simulink library "kalmanlib"  (Simulink 7.0)
undefined symbols (not defined in the file): dt, P0, Q, seed1, tS, x0
libraries: kalmanlib x10, simulink x6
(part 1 of 2)
settings Model: Creator=peter  LastModifiedBy=peter  ExtModeAutoUpdateStatusClock=off

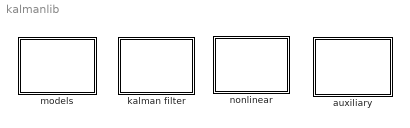
== system kalmanlib ==
  auxiliary : Subsystem
  kalman filter : Subsystem
  models : Subsystem
  nonlinear : Subsystem

== system kalmanlib/auxiliary ==
  Discrete Derivative : Subsystem  mask{x0=1, tS=0.01}
      mask prompts: x0 "Anfangs-Wert für x"; tS "Sample-Zeit"
      mask Display:
      | port_label('input', 1, 'x')
      | port_label('output', 1, 'v')
      | text(0.4, 0.7, 'd')
      | text(0.4, 0.4, 'dt')
      | plot([0.35 0.6], [0.5 0.5])
  Mean : Subsystem  mask{tS=1}
      mask prompts: tS "Sample-Zeit"
      mask Display: disp('total mean\n over time')
  Multivariate Normal  Distribution : Subsystem  mask(Multivariate Normal Distribution){m=0, P=Q, seed=seed1, tS=tS, C=0}
      mask prompts: m "Mean"; P "Covariance matrix"; seed "Initial seed"; tS "Sample time"; C "Root of P"
      mask help: Output a multivariate normally (Gaussian) distributed random signal.
      mask init:
      | [C, res] = sqrtm(P);
      mask Display: disp('N(m,P)')
  Osci : Subsystem
      settings: OpenFcn=open_system(find_system(gcbh, 'Name', 'Scope'), 'force')
  Variable Multivariate  Normal Distribution : Subsystem  mask(Multivariate Normal Distribution){m=0, seed=seed', tS=dt}
      mask prompts: m "Mean"; seed "Initial seed"; tS "Sample time"
      mask help: Output a multivariate normally (Gaussian) distributed random signal.
      mask Display:
      | port_label('input', 1, 'P')
      | port_label('output', 1, 'N(m,P)')

== system kalmanlib/kalman filter ==
  Extended Kalman Filter (Measurement) : Subsystem  mask(Kalman Filter){A=[1, 0, 1, 0, 0.5, 0; 0, 1, 0, 1, 0, 0.5;   0, 0, 1, 0, 1, 0; 0, 0, 0, 1, 0, 1;  0, 0, 0, 0, 1, 0;  0, 0, 0, 0, 0, 1], B=0, Q=[1 0 2 0 2 0; 0 1 0 2 0 2; 2 0 4 0 4 0; 0 2 0 4 0 4; 2 0 4 0 4 0; 0 2 0 4 0 4]*1e-4, R=[4 0; 0 4]*1e-4, x0=[40.254 25.117 0.492 0.112 -0.02 0.02]', P0=diag([100 100 1 1 0 0])*1e-6}
      mask prompts: A "Übertragungsmatrix A"; B "Kontrollmatrix B"; Q "Varianz der x-Störung Q"; R "Varianz der y-Störung R"; x0 "geschätzter Anfangsvektor x0"; P0 "geschätzte x-Anfangsvarianz P"
      mask Display:
      | disp('EKF (M)')
      | port_label('input', 1, 'u')
      | port_label('input', 2, 'z')
      | port_label('output', 1, 'x')
      | port_label('output', 2, 'P')
  Extended Kalman Filter (System) : Subsystem  mask(Extended Kalman Filter (A)){B=0, H=[1,0,0], Q=[0 0 0; 0 0 0; 0 0 0], R=[1e-3], x0=[1; 0; 0], P0=[1,0,0; 0,1,0; 0,0,10]*1e-2}
      mask prompts: B "Kontrollmatrix B"; H "Beobachtungsmatrix H"; Q "Varianz der x-Störung Q"; R "Varianz der y-Störung R"; x0 "geschätzter Anfangsvektor x0"; P0 "geschätzte x-Anfangsvarianz P"
      mask help: Extended Kalman Filter with a nonlinear system block, but linear control and measurement
      mask Display:
      | disp('EKF (A)')
      | port_label('input', 1, 'u')
      | port_label('input', 2, 'z')
      | port_label('output', 1, 'x')
      | port_label('output', 2, 'P')
  Kalman Filter : Subsystem  mask(Kalman Filter){A=[cos(0.01), sin(0.01); -sin(0.01), cos(0.01)], B=0, H=[1,0], Q=[0 0; 0 0], R=[2e-4], x0=[1; 0], P0=[10, 0; 0, 10]*1e-3}
      mask prompts: A "system matrix A"; B "control matrix B"; H "observation matrix H"; Q "variance of system noise Q"; R "variance of  measurement noise R"; x0 "estimated initial value x0"; P0 "estimated initial filter variance P0"
      mask Display:
      | disp('KF')
      | port_label('input', 1, 'u')
      | port_label('input', 2, 'z')
      | port_label('output', 1, 'x')
      | port_label('output', 2, 'P')
  "Kalman Filter A(t), Q(t), B(t) H(t), R(t)" : Subsystem  mask(Kalman Filter){x0=x0, P0=P0}
      mask prompts: x0 "geschätzter Anfangsvektor x0"; P0 "geschätzte x-Anfangsvarianz P"
      mask help: Kalman Filter with complete time-dependent system matrices A(t), Q(t), controll matrix B(t) and measurement matrices H(t), R(t)
      mask Display:
      | disp('KF\nA(t),M(t)')
      | port_label('input', 1, 'u')
      | port_label('input', 2, 'z')
      | port_label('input', 3, 'A')
      | port_label('input', 4, 'Q')
      | port_label('input', 5, 'B')
      | port_label('input', 6, 'H')
      | port_label('input', 7, 'R')
      | port_label('output', 1, 'x')
      | port_label('output', 2, 'P')
  "Kalman Filter Akin, H(t), R(t)" : Subsystem  mask(Kalman Filter){q=1e-3, x0=[0; 0; 0], P0=[1,0,0; 0,1,0; 0,0,100]*1e-3}
      mask prompts: q "Varianz der Systembeschleunigung"; x0 "geschätzter Anfangsvektor x0"; P0 "geschätzte x-Anfangsvarianz P0"
      mask help: Kalman filter with kinematical model, no control input and time dependent measurement matrices
      mask Display:
      | disp('KF\nAkin,M(t)')
      | port_label('input', 1, 'z')
      | port_label('input', 2, 'H')
      | port_label('input', 3, 'R')
      | port_label('output', 1, 'x')
      | port_label('output', 2, 'P')
  "Kalman Filter H(t), R(t)" : Subsystem  mask(Kalman Filter){A=[cos(0.01), sin(0.01); -sin(0.01), cos(0.01)], B=0, Q=[1 0; 0 1]*1e-5, x0=[1; 0], P0=[10, 0; 0, 10]*1e-3}
      mask prompts: A "Übertragungsmatrix A"; B "Kontrollmatrix B"; Q "Varianz der x-Störung Q"; x0 "geschätzter Anfangsvektor x0"; P0 "geschätzte x-Anfangsvarianz P"
      mask Display:
      | disp('KF\n(M(t))')
      | port_label('input', 1, 'u')
      | port_label('input', 2, 'z')
      | port_label('input', 3, 'H')
      | port_label('input', 4, 'R')
      | port_label('output', 1, 'x')
      | port_label('output', 2, 'P')

== system kalmanlib/models ==
  1d Measurement : Subsystem  mask(1d Measurement){z=[0.1380,0.0910,-0.0159,-0.0136,-0.0077,0.0439,0.2266,0.1905,0.1482,0.2501,0.2176,0.1823,0.2939,0.2124,0.2453,0.2628,0.2903,0.3583,0.4089,0.1523,0.3729,0.3517,0.2519,0.4215,0.3956,0.3202,0.3627,0.3605,0.2716,0.2636,0.1681,0.2734,0.2175,0.2250,0.1503,0.2735,0.2233,0.1984,0.2355,0.1392,0.2024,0.2602,0.0327,0.0900,0.1105,0.0045,0.0430,0.0364,0.0511,-0.0794,-0.0481,0.0757,0.0581,0.0242,-0.0072,0.0637,-0.0470,0.0910,0.0288,0.0613,0.0959,0.0072,0.0347,0.0589,0.0567,0.0587,0.0188,-0.1641,-0.1057,0.0336,0.0292,-0.0035,0.0348,0.0015,-0.0945,0.0757,-0.0804,0.0287,0.0560,0.0164,-0.0787,-0.0633,0.0008,-0.0201,0.0182,0.0780,-0.0259,-0.0030,0.0018,-0.0071,-0.0517,0.0320,-0.0405,0.1683,-0.0485,-0.0216,0.1008,0.0645,0.1713,0.0181,-0.0610,0.0059,0.0245,0.0179,0.0479,0.0177,0.0540,-0.0117,0.1367,0.0155,0.0139,-0.0703,0.0292,0.0298,-0.0299,-0.1043,-0.0009,-0.1086,0.0372,-0.0380,-0.0583,0.0088,0.1045,-0.0563,0.0079,0.0523,-0.0700,-0.0429,-0.0003,-0.0805,0.0107,0.0343,0.0600,-0.0270,-0.0023,-0.0242,-0.0833,-0.0319,-0.0474,-0.0524,0.0017,0.0226,0.1168,-0.0347,-0.0742,-0.0482,0.0680,0.0178,-0.0728,-0.0572,0.0243,0.1647,-0.0901,-0.0689,0.1284,-0.0018,0.0460,0.1346,0.0367,0.0288,-0.0522,0.1281,0.0547,-0.1040,0.0695,-0.0124,0.1157,-0.0386,-0.0906,-0.0311,-0.0158,-0.0269,0.0090,-0.0282,0.0973,-0.0211,0.0469,0.0129,-0.0029,0.0412,0.0162,-0.0218,0.0834,0.0718,0.1081,-0.0991,0.0362,0.0191,0.0636,-0.0240,0.0211,0.0351,0.0912,0.0355,-0.0504,0.0776,-0.0542,-0.0138,-0.0517,0.0402,-0.0159,-0.0693,-0.0044,-0.0406,0.0775,-0.0301,0.0169,-0.1656,0.0031,-0.0002,-0.0002,-0.0222,0.0299,0.0839,0.0432,0.0390,0.1020,-0.0606,-0.0225,-0.0315,0.0205,-0.0384,0.0609,0.0658,0.0217,-0.0621,0.1851,-0.0227,0.0892,-0.0574,-0.0949,-0.0608,-0.0221,-0.1220,0.0377,-0.0256,-0.1393,0.0241,0.0745,0.0055,-0.0394,0.0414,-0.0244,-0.0742,-0.1368,-0.1062,0.1675,0.0669,0.1247,0.0141,-0.0024,0.0408,0.1104,0.0527,0.0211,0.0818,-0.0051,0.0152,-0.0720,0.0521,-0.0437,-0.1017,-0.0702,-0.0770,0.0094,0.0270,0.0268,0.0822,-0.0898,-0.0408,-0.0599,-0.0616,0.0117,-0.0002,-0.0380,0.0367,-0.0361,0.0682,0.0739,0.1148,-0.0767,0.0196,-0.0155,-0.0191,-0.0290,0.0401,-0.0479,-0.0988,-0.0381,-0.0880,-0.0745,-0.0173,-0.1304,-0.0234,0.0113,0.0536,0.1192,-0.0779,0.0781,0.0205,-0.0492,0.0340,0.1151,-0.0780,-0.0607,0.0280,-0.0513,-0.0101,-0.0150,-0.1015,-0.0016,-0.1662,-0.1473,0.0174,-0.0300,-0.0059,0.0527,0.0109,-0.0536,0.0899,0.0172,-0.0751,0.0311,0.0188,0.0247,-0.0393,-0.0340,0.0261,-0.0992,0.0299,0.0613,-0.0295,0.0995,-0.0635,-0.1087,-0.0616,-0.0558,-0.1064,-0.0866,-0.1732,-0.1533,-0.2250,-0.0651,-0.1563,-0.1172,-0.1588,-0.1073,-0.1476,-0.1861,-0.1991,-0.1407,-0.2104,-0.2448,-0.3369,-0.2338,-0.1268,-0.2679,-0.2480,-0.2131,-0.3307,-0.2384,-0.2872,-0.2326,-0.1490,-0.3296,-0.2361,-0.1340,-0.2121,-0.1659,-0.2511,-0.2221,-0.2425,-0.1999,-0.3223,-0.2122,-0.2645,-0.2355,-0.1476,-0.1370,-0.1293,-0.1295,-0.1347,-0.1724,-0.2233,-0.1083,-0.2197,-0.2449,-0.2328,-0.0774,-0.1419,-0.0486,-0.1217,0.0140,-0.0769,-0.0736,-0.0718,-0.0677,-0.1021,-0.0398,0.0411,0.0987,0.0298,-0.0053,-0.0568,0.0283,0.0070,0.0412,-0.1630,0.0166,0.0811,0.0049,-0.0100,0.0485,0.0776,-0.0413,0.0282,-0.0217,-0.0693,0.0684,-0.0315,-0.0507,0.0911,-0.0213,0.0048,-0.0687,0.0454,-0.0290,-0.1052,0.0866,-0.0460,0.0028,-0.0073,-0.0241,0.0642,0.0418,0.0690,0.0297,-0.0614,0.0997,-0.0041,0.0422,-0.0466,0.0158,-0.0483,-0.0694,0.0159,-0.0469,-0.0427,0.0806,-0.0196,0.0309], tS=1}
      mask prompts: z "measurement values"; tS "sample time"
      mask help: outputs a given list of one-dimensional measurement values
      mask Display: plot(1:size(z,2), z)
  2d Measurement : Subsystem  mask(2d Measurement){zx=[1 2 3 2 1], zy=[0 1 0 -1 0], tS=1}
      mask prompts: zx "Messwerte, x-Komponente"; zy "Messwerte, y-Komponente"; tS "Sample-Zeit"
      mask help: outputs a given list of two-dimensional measurement values
      mask Display:
      | port_label('output', 1, 'z')
      | plot(zx, zy)
  Damped Oscillator : Subsystem  mask(DampedOscillator){omega0=2, D=0.1, x0=1, v0=0, dt=0.1, R=0.1, seed=1}
      mask prompts: omega0 "angular frequency"; D "damping coefficient"; x0 "initial displacement"; v0 "initial velocity"; dt "sample time"; R "variance of measurement"; seed "initial seed"
      mask help:
      | Linear oscillator with harmonic damping
      | u:  control input
      | x: system output (x, v)
      | y: measurement output (x + W)
      mask Display:
      | plot([0:0.2:5], [1.0000,0.8321,0.4092,-0.1005,
      |      -0.5195,-0.7201,-0.6610,-0.3910,-0.0228,0.3113,
      |      0.5051,0.5107,0.3476,0.0885,-0.1705,-0.3440,
      |      -0.3847,-0.2941,-0.1170,0.0786,0.2262,0.2827,
      |      0.2397,0.1227,-0.0215,-0.1423])
      | port_label('input', 1, 'u')
      | port_label('output', 1, 'x')
      | port_label('output', 2, 'z')
  Damped Oscillator3 : Subsystem  mask(DampedOscillator3){omega0=2, D=0.2, x0=1, v0=0, dt=0.01, R=1e-3, seed=1}
      mask prompts: omega0 "angular frequency"; D "damping coefficient"; x0 "initial displacement"; v0 "initial velocity"; dt "sample time"; R "variance of measurement"; seed "initial seed"
      mask help:
      | Linear oscillator with harmonic damping and additional output of the damping ration D
      | u:  control input
      | x: system output (x, v, D)
      | y: measurement output (x + W)
      mask Display:
      | plot([0:0.2:5], [1.0000,0.8321,0.4092,-0.1005,
      |      -0.5195,-0.7201,-0.6610,-0.3910,-0.0228,0.3113,
      |      0.5051,0.5107,0.3476,0.0885,-0.1705,-0.3440,
      |      -0.3847,-0.2941,-0.1170,0.0786,0.2262,0.2827,
      |      0.2397,0.1227,-0.0215,-0.1423])
      | port_label('input', 1, 'u')
      | port_label('output', 1, 'x')
      | port_label('output', 2, 'z')
  Flight1d : Subsystem  mask(Flight1D){tS=50, tF=280, tL=70, v0=10, q=0.001, dt=1, seed=17}
      mask prompts: tS "duration of start"; tF "duration of cruise"; tL "duration of landing"; v0 "cruise velocity"; q "variance of acceleration"; dt "sample time"; seed "initial seed"
      mask Display:
      | plot([1:6,18:26],
      |      [0,0.97,3.49,6.57,9.02,10.0,10.0,9.60,
      |       8.28,6.25,4.06,2.10,0.72,0.26,0.28])
      | port_label('output', 1, 'x')
  Harmonic Oscillator : Subsystem  mask(Discrete harmonic oscillator){w=4, x0=0, v0=0, R=2e-4, seed=0, dt=0.05}
      mask prompts: w "angular frequency"; x0 "initial displacement"; v0 "initial velocity"; R "variance of measurement"; seed "initial seed"; dt "sample time"
      mask Display:
      | plot(0:0.1:2*pi,sin(0:0.1:2*pi))
      | port_label('input', 1, 'u')
      | port_label('output', 1, 'x')
      | port_label('output', 2, 'z')
  Harmonic Oszillator (cont.) : Subsystem  mask(Harmonic oscillator){omega0=1, x0=1, v0=0, R=2e-4, seed=0, dt=0.01}
      mask prompts: omega0 "angular frequency"; x0 "initial displacement"; v0 "initial velocity"; R "variance of measurement"; seed "initial seed"; dt "sample time"
      mask help:
      | Linear oscillator
      | u:  control input
      | x: system output (x, v)
      | y: measurement output (x + W)
      mask Display:
      | plot(0:0.1:2*pi,sin(0:0.1:2*pi))
      | port_label('input', 1, 'u')
      | port_label('output', 1, 'x')
      | port_label('output', 2, 'z')
  Linear Measurement : Subsystem  mask(LinearMeasurement){H=[0 0 1], R=0.003, dt=1, seed=43}
      mask prompts: H "observation matrix"; R "variance of measurement"; dt "sample time"; seed "initial seed"
      mask Display:
      | port_label('input', 1, 'x')
      | port_label('output', 1, 'z')
      | 
      | plot([0.15 0.85], [0.53 0.53])
      | plot([0.15 0.85], [0.47 0.47])
  Linear System : Subsystem  mask(Linear System with Noise){A=[0.9950, 0.0998; -0.0998, 0.9950], B=0, H=[1, 0], Q=[0 0; 0 0], R=2e-2, x0=[1; 0], tS=0.05, seed=17}
      mask prompts: A "system matrix A"; B "control matrix B"; H "observation matrix H"; Q "variance of system noise Q"; R "variance of  measurement noise R"; x0 "initial value x0"; tS "sample time"; seed "initial seed"
      mask help:
      | Linear System with Gaussian Noise given by
      |   x(k+1) = A x(k) + B u(k) + w(k)
      |   y(k) = H x(k) + v(k)
      | w(k), v(k) are Gaussian random variables with mean 0 and variance Q, R
      mask init:
      | N = size(Q, 1);
      | M = size(R, 1);
      | seed1 = (seed:(seed+N-1))';
      | seed2 = ((seed+N):(seed+N+M-1))';
      mask Display:
      | text(0.15, 0.65, 'x_{k+1} = Ax_k+Bu_k+w_k',
      |   'texmode', 'on', 'horizontalAlignment', 'left')
      | text(0.15, 0.35, 'z_k = Hx_k+v_k',
      |   'texmode', 'on', 'horizontalAlignment', 'left')
      | port_label('output', 1, 'x')
      | port_label('output', 2, 'z')
      | port_label('input', 1, 'u')
  Two-Phase Measurement : Subsystem  mask(TwoPhaseMeasurement){H1=[0 0 1; 0 0 0], H2=[0 0 1; 1 0 0], R1=[0.003, 0; 0, 1e-10], R2=[0.003, 0; 0, 1], n=100, dt=0.1, seed=[43,28]}
      mask prompts: H1 "observation matrix H1"; H2 "observation matrix H2"; R1 "variance of measurement R1"; R2 "variance of measurement R2"; n "decimation factor n of measurement 2"; dt "sample time dt"; seed "initial seed"
      mask help:
      | combination of two measurements:
      | - usual measurements are given by H1, R1
      |    samples are taken each dt
      | - every n'th sample is taken using H2, R2 instead
      mask Display:
      | port_label('input', 1, 'x')
      | port_label('output', 1, 'z')
      | port_label('output', 2, 'H')
      | port_label('output', 3, 'R')
      | 
      | plot([0.15 0.5 0.5 0.85], [0.53 0.53 0.87 0.87])
      | plot([0.15 0.55 0.55 0.85], [0.47 0.47 0.8 0.8])

== system kalmanlib/nonlinear ==
  2-Point-Distance : Subsystem  mask(twoPointDistance){P1=[1000;4000], P2=[3000;0], R=[1 0; 0 1]*0000, dt=1, seed=[1 2]'}
      mask prompts: P1 "1. Bezugspunkt"; P2 "2. Bezugspunkt"; R "variance of  measurement noise R"; dt "sample time"; seed "initial seed"
      mask help:
      | Measurement z = h(x) given by the distance to two fixed points P1, P2.
      | Assumes input vector of the form (x, y, vx, vy, ax, ay).
      |
      | returns h(x) and the Jacobi Matrix H
  Damped Oscillator3 (Lin.) : Subsystem
      mask Type: dampedOscillatorLin2
      mask Description:
      | Model x_k = f(x_{k-1}) of a damped oscillator. The state vector x is augmented by the damping ratio D:
      |    xvec = (x, v, D)
      | f(x) is a sampled version of the real dynamics.
      | Additionally returns the Jacobi Matrix A.
  Damped Oscillator3 (Lin.) 1-st order : Subsystem
      mask Type: dampedOscillatorLin1
      mask Description:
      | Model x_k = f(x_{k-1}) of a damped oscillator in 1st order. The state vector x is augmented by the damping ratio D:
      |    xvec = (x, v, D)
      | f(x) is an Euler approximation of the real dynamics.
      | Additionally returns the Jacobi Matrix A.

== system kalmanlib/auxiliary/Discrete Derivative ==
  In1 : Inport  OutDataType=sfix(16)  OutScaling=2^0
  Gain : Gain  Gain=1/tS  ParameterDataType=sfix(16)  ParameterScaling=2^0  OutDataType=sfix(16)  OutScaling=2^0
  Sum : Sum  Inputs=|+-  OutDataType=sfix(16)  OutScaling=2^0
  Unit Delay : UnitDelay  X0=x0  SampleTime=-1
  Out1 : Outport  OutDataType=sfix(16)  OutScaling=2^0
  wires:
  In1/1 -> Unit Delay/1, Sum/1
  Unit Delay/1 -> Sum/2
  Sum/1 -> Gain/1
  Gain/1 -> Out1/1

== system kalmanlib/auxiliary/Mean ==
  note: prevents division
      |  by 0 at startup
  In1 : Inport  OutDataType=sfix(16)  OutScaling=2^0
  Bias : Bias  Bias=eps
  Clock : Clock
  Divide : Product  Inputs=*/  OutDataType=sfix(16)  OutScaling=2^-10
  Gain1 : Gain  Gain=1/tS  ParameterDataType=sfix(16)  ParameterScaling=2^0  OutDataType=sfix(16)  OutScaling=2^0
  Sum : Sum  Inputs=|++  OutDataType=sfix(16)  OutScaling=2^0
  Unit Delay : UnitDelay  SampleTime=-1
  Zero-Order Hold : ZeroOrderHold  SampleTime=tS
  Out1 : Outport  OutDataType=sfix(16)  OutScaling=2^0
  wires:
  Bias/1 -> Divide/2
  Gain1/1 -> Bias/1
  Zero-Order Hold/1 -> Out1/1
  Divide/1 -> Zero-Order Hold/1
  In1/1 -> Sum/1
  Sum/1 -> Unit Delay/1
  Unit Delay/1 -> Divide/1, Sum/2
  Clock/1 -> Gain1/1

== system kalmanlib/auxiliary/Multivariate Normal  Distribution ==
  Bias : Bias  Bias=m
  Gain : Gain  Gain=C  Multiplication=Matrix(K*u)  ParameterDataType=sfix(16)  ParameterScaling=2^0  OutDataType=sfix(16)  OutScaling=2^0
  Random Number : RandomNumber  Seed=seed  SampleTime=tS  VectorParams1D=off
  Out1 : Outport  OutDataType=sfix(16)  OutScaling=2^0
  wires:
  Bias/1 -> Out1/1
  Gain/1 -> Bias/1
  Random Number/1 -> Gain/1

== system kalmanlib/auxiliary/Osci ==
  x : Inport  OutDataType=sfix(16)  OutScaling=2^0
  z : Inport  Port=2  OutDataType=sfix(16)  OutScaling=2^0
  xKF : Inport  Port=3  OutDataType=sfix(16)  OutScaling=2^0
  p : Inport  Port=4  OutDataType=sfix(16)  OutScaling=2^0
  Abs : Abs
  MATLAB Fcn : MATLABFcn  MATLABFcn=diag(u)
  Math Function : Math  Operator=sqrt  OutDataType=sfix(16)  OutScaling=2^0  SaturateOnIntegerOverflow=on
  Scope : Scope  NumInputPorts=5
      settings: TimeRange=700  YMin=-1000~-0.5~-1000~0~0  YMax=5000~0.5~5000~600~400
  Sum : Sum  Inputs=+-|  OutDataType=sfix(16)  OutScaling=2^0
  wires:
  MATLAB Fcn/1 -> Math Function/1
  Math Function/1 -> Scope/4  "filter sigma"
  Sum/1 -> Abs/1
  Abs/1 -> Scope/5  "error"
  x/1 -> Scope/1, Sum/2  "x from system"
  z/1 -> Scope/2  "measurement"
  xKF/1 -> Scope/3, Sum/1  "x from filter"
  p/1 -> MATLAB Fcn/1

== system kalmanlib/auxiliary/Variable Multivariate  Normal Distribution ==
  R : Inport  OutDataType=sfix(16)  OutScaling=2^0
  Bias : Bias  Bias=m
  MATLAB Fcn : MATLABFcn  MATLABFcn=sqrtm(u)  Output1D=off
  Product : Product  Multiplication=Matrix(*)  OutDataType=sfix(16)  OutScaling=2^0  RndMeth=Zero
  Random Number : RandomNumber  Seed=seed  SampleTime=tS  VectorParams1D=off
  Out1 : Outport  OutDataType=sfix(16)  OutScaling=2^0
  wires:
  Random Number/1 -> Product/2
  MATLAB Fcn/1 -> Product/1
  Product/1 -> Bias/1
  Bias/1 -> Out1/1
  R/1 -> MATLAB Fcn/1

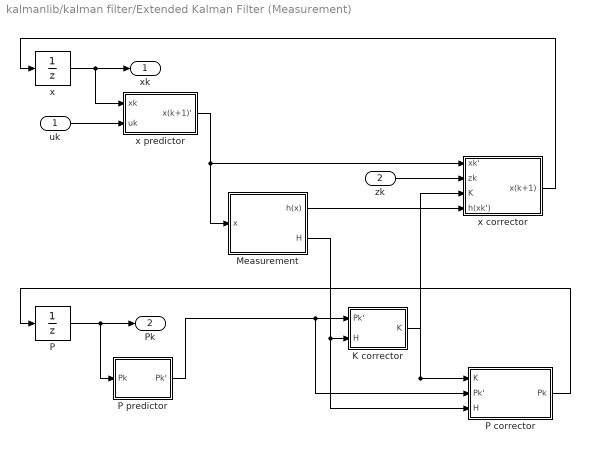
== system kalmanlib/kalman filter/Extended Kalman Filter (Measurement) ==
  uk : Inport  OutDataType=sfix(16)  OutScaling=2^0
  zk : Inport  Port=2  OutDataType=sfix(16)  OutScaling=2^0
  K corrector : Subsystem
  Measurement : Subsystem
  P : UnitDelay  X0=P0  SampleTime=-1
  P corrector : Subsystem
  P predictor : Subsystem
  x : UnitDelay  X0=x0  SampleTime=-1
  x corrector : Subsystem
  x predictor : Subsystem
  xk : Outport  OutDataType=sfix(16)  OutScaling=2^0
  Pk : Outport  Port=2  OutDataType=sfix(16)  OutScaling=2^0
  wires:
  Measurement/2(H) -> P corrector/3(H), K corrector/2(H)
  Measurement/1(h(x)) -> x corrector/4(h(xk'))
  x corrector/1(x(k+1)) -> x/1
  x/1 -> x predictor/1(xk), xk/1
  P corrector/1(Pk) -> P/1
  K corrector/1(K) -> P corrector/1(K), x corrector/3(K)
  P predictor/1(Pk') -> K corrector/1(Pk'), P corrector/2(Pk')
  P/1 -> Pk/1, P predictor/1(Pk)
  x predictor/1(x(k+1)') -> x corrector/1(xk'), Measurement/1(x)
  zk/1 -> x corrector/2(zk)
  uk/1 -> x predictor/2(uk)

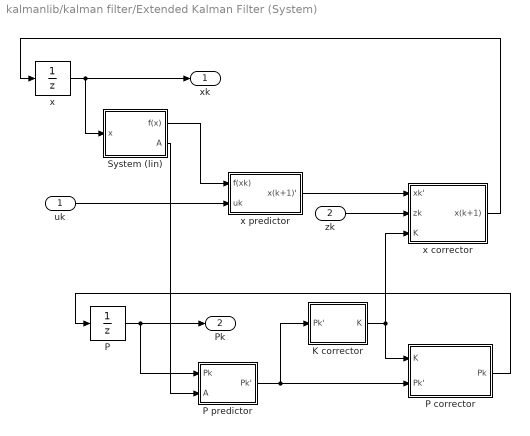
== system kalmanlib/kalman filter/Extended Kalman Filter (System) ==
  uk : Inport  OutDataType=sfix(16)  OutScaling=2^0
  zk : Inport  Port=2  OutDataType=sfix(16)  OutScaling=2^0
  K corrector : Subsystem
  P : UnitDelay  X0=P0  SampleTime=-1
  P corrector : Subsystem
  P predictor : Subsystem
  System (lin) : Subsystem
  x : UnitDelay  X0=x0  SampleTime=-1
  x corrector : Subsystem
  x predictor : Subsystem
  xk : Outport  OutDataType=sfix(16)  OutScaling=2^0
  Pk : Outport  Port=2  OutDataType=sfix(16)  OutScaling=2^0
  wires:
  System (lin)/2(A) -> P predictor/2(A)
  System (lin)/1(f(x)) -> x predictor/1(f(xk))
  uk/1 -> x predictor/2(uk)
  zk/1 -> x corrector/2(zk)
  x predictor/1(x(k+1)') -> x corrector/1(xk')
  P/1 -> P predictor/1(Pk), Pk/1
  P predictor/1(Pk') -> P corrector/2(Pk'), K corrector/1(Pk')
  K corrector/1(K) -> x corrector/3(K), P corrector/1(K)
  P corrector/1(Pk) -> P/1
  x/1 -> System (lin)/1(x), xk/1
  x corrector/1(x(k+1)) -> x/1

== system kalmanlib/kalman filter/Kalman Filter ==
  uk : Inport  OutDataType=sfix(16)  OutScaling=2^0
  zk : Inport  Port=2  OutDataType=sfix(16)  OutScaling=2^0
  K corrector : Subsystem
  P : UnitDelay  X0=P0  SampleTime=-1
  P corrector : Subsystem
  P predictor : Subsystem
  x : UnitDelay  X0=x0  SampleTime=-1
  x corrector : Subsystem
  x predictor : Subsystem
  xk : Outport  OutDataType=sfix(16)  OutScaling=2^0
  Pk : Outport  Port=2  OutDataType=sfix(16)  OutScaling=2^0
  wires:
  uk/1 -> x predictor/2(uk)
  zk/1 -> x corrector/2(zk)
  x predictor/1(x(k+1)') -> x corrector/1(xk')
  P/1 -> P predictor/1(Pk), Pk/1
  P predictor/1(Pk') -> P corrector/2(Pk'), K corrector/1(Pk')
  K corrector/1(K) -> x corrector/3(K), P corrector/1(K)
  P corrector/1(Pk) -> P/1
  x/1 -> xk/1, x predictor/1(xk)
  x corrector/1(x(k+1)) -> x/1

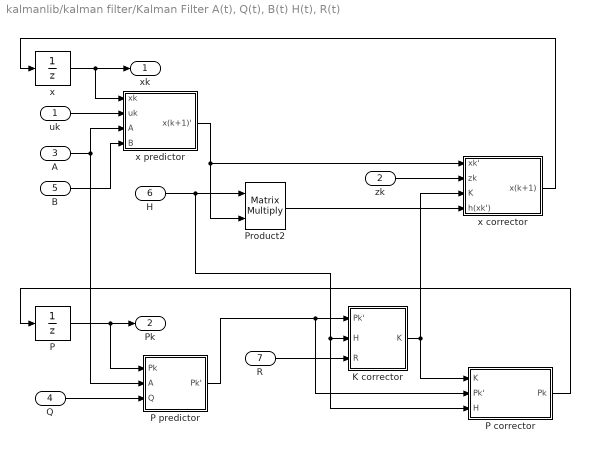
== system kalmanlib/kalman filter/Kalman Filter A(t), Q(t), B(t) H(t), R(t) ==
  uk : Inport  OutDataType=sfix(16)  OutScaling=2^0
  zk : Inport  Port=2  OutDataType=sfix(16)  OutScaling=2^0
  A : Inport  Port=3  OutDataType=sfix(16)  OutScaling=2^0
  Q : Inport  Port=4  OutDataType=sfix(16)  OutScaling=2^0
  B : Inport  Port=5  OutDataType=sfix(16)  OutScaling=2^0
  H : Inport  Port=6  OutDataType=sfix(16)  OutScaling=2^0
  R : Inport  Port=7  OutDataType=sfix(16)  OutScaling=2^0
  K corrector : Subsystem
  P : UnitDelay  X0=P0  SampleTime=-1
  P corrector : Subsystem
  P predictor : Subsystem
  Product2 : Product  Multiplication=Matrix(*)  OutDataType=sfix(16)  OutScaling=2^0  RndMeth=Zero
  x : UnitDelay  X0=x0  SampleTime=-1
  x corrector : Subsystem
  x predictor : Subsystem
  xk : Outport  OutDataType=sfix(16)  OutScaling=2^0
  Pk : Outport  Port=2  OutDataType=sfix(16)  OutScaling=2^0
  wires:
  B/1 -> x predictor/4(B)
  Q/1 -> P predictor/3(Q)
  A/1 -> P predictor/2(A), x predictor/3(A)
  uk/1 -> x predictor/2(uk)
  zk/1 -> x corrector/2(zk)
  x predictor/1(x(k+1)') -> x corrector/1(xk'), Product2/2
  P/1 -> P predictor/1(Pk), Pk/1
  P predictor/1(Pk') -> P corrector/2(Pk'), K corrector/1(Pk')
  K corrector/1(K) -> x corrector/3(K), P corrector/1(K)
  P corrector/1(Pk) -> P/1
  x/1 -> xk/1, x predictor/1(xk)
  x corrector/1(x(k+1)) -> x/1
  Product2/1 -> x corrector/4(h(xk'))
  H/1 -> Product2/1, K corrector/2(H), P corrector/3(H)
  R/1 -> K corrector/3(R)

== system kalmanlib/kalman filter/Kalman Filter Akin, H(t), R(t) ==
  z : Inport  OutDataType=sfix(16)  OutScaling=2^0
  H : Inport  Port=2  OutDataType=sfix(16)  OutScaling=2^0
  R : Inport  Port=3  OutDataType=sfix(16)  OutScaling=2^0
  B : Constant  Value=0  VectorParams1D=off  OutDataType=sfix(16)  OutScaling=2^0
  Ground1 : Ground
  "Kalman Filter A(t), Q(t), B(t) H(t), R(t)" : kalmanlib/kalman filter/Kalman Filter A(t), Q(t), B(t) H(t), R(t)  SystemSampleTime=-1  x0=x0  P0=P0
  MATLAB Fcn : MATLABFcn  MATLABFcn=[1, u, 0.5*u^2; 0, 1, u; 0, 0, 1]  Output1D=off
  MATLAB Fcn1 : MATLABFcn  MATLABFcn=[0.050*u^5,0.125*u^4,0.167*u^3; 0.125*u^4,0.333*u^3,0.500*u^2; 0.167*u^3,0.500*u^2,1.000*u]*q  Output1D=off
  Weighted Sample Time : simulink/Math Operations/Weighted Sample Time Math  TsampMathOp=Ts Only  weightValue=1.0  TsampMathImp=Online Calculations  DoSatur=off
  x : Outport  OutDataType=sfix(16)  OutScaling=2^0
  P : Outport  Port=2  OutDataType=sfix(16)  OutScaling=2^0
  wires:
  Ground1/1 -> "Kalman Filter A(t), Q(t), B(t) H(t), R(t)"/1
  "Kalman Filter A(t), Q(t), B(t) H(t), R(t)"/1 -> x/1
  "Kalman Filter A(t), Q(t), B(t) H(t), R(t)"/2 -> P/1
  z/1 -> Weighted Sample Time/1, "Kalman Filter A(t), Q(t), B(t) H(t), R(t)"/2
  H/1 -> "Kalman Filter A(t), Q(t), B(t) H(t), R(t)"/6
  R/1 -> "Kalman Filter A(t), Q(t), B(t) H(t), R(t)"/7
  B/1 -> "Kalman Filter A(t), Q(t), B(t) H(t), R(t)"/5
  MATLAB Fcn/1 -> "Kalman Filter A(t), Q(t), B(t) H(t), R(t)"/3
  MATLAB Fcn1/1 -> "Kalman Filter A(t), Q(t), B(t) H(t), R(t)"/4
  Weighted Sample Time/1 -> MATLAB Fcn/1, MATLAB Fcn1/1

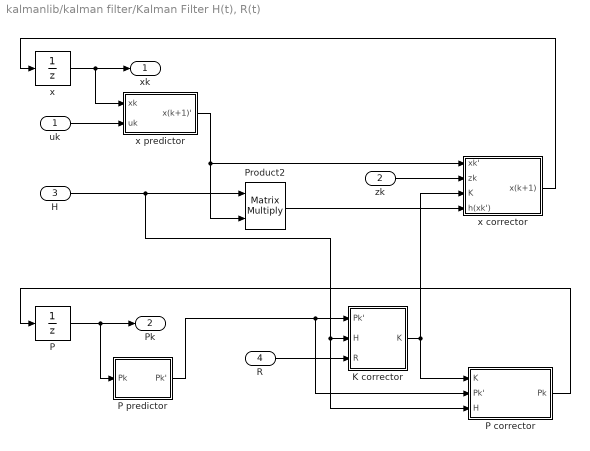
== system kalmanlib/kalman filter/Kalman Filter H(t), R(t) ==
  uk : Inport  OutDataType=sfix(16)  OutScaling=2^0
  zk : Inport  Port=2  OutDataType=sfix(16)  OutScaling=2^0
  H : Inport  Port=3  OutDataType=sfix(16)  OutScaling=2^0
  R : Inport  Port=4  OutDataType=sfix(16)  OutScaling=2^0
  K corrector : Subsystem
  P : UnitDelay  X0=P0  SampleTime=-1
  P corrector : Subsystem
  P predictor : Subsystem
  Product2 : Product  Multiplication=Matrix(*)  OutDataType=sfix(16)  OutScaling=2^0  RndMeth=Zero
  x : UnitDelay  X0=x0  SampleTime=-1
  x corrector : Subsystem
  x predictor : Subsystem
  xk : Outport  OutDataType=sfix(16)  OutScaling=2^0
  Pk : Outport  Port=2  OutDataType=sfix(16)  OutScaling=2^0
  wires:
  R/1 -> K corrector/3(R)
  H/1 -> P corrector/3(H), K corrector/2(H), Product2/1
  Product2/1 -> x corrector/4(h(xk'))
  x corrector/1(x(k+1)) -> x/1
  x/1 -> x predictor/1(xk), xk/1
  P corrector/1(Pk) -> P/1
  K corrector/1(K) -> P corrector/1(K), x corrector/3(K)
  P predictor/1(Pk') -> K corrector/1(Pk'), P corrector/2(Pk')
  P/1 -> Pk/1, P predictor/1(Pk)
  x predictor/1(x(k+1)') -> Product2/2, x corrector/1(xk')
  zk/1 -> x corrector/2(zk)
  uk/1 -> x predictor/2(uk)

== system kalmanlib/models/1d Measurement ==
  Clock : Clock
      settings: Decimation=10
  Compare To Constant : simulink/Logic and Bit Operations/Compare To Constant  SystemSampleTime=-1  relop=>=  const=size(z,2)*tS  LogicOutDataTypeMode=boolean  ZeroCross=off
  Lookup Table : Lookup  InputValues=(0:(size(z,2)-1))*tS  Table=z'  LookUpMeth=Interpolation-Use End Values  OutDataType=sfix(16)  OutScaling=2^0  SampleTime=tS
  Stop Simulation : Stop
  Out1 : Outport  OutDataType=sfix(16)  OutScaling=2^0
  wires:
  Compare To Constant/1 -> Stop Simulation/1
  Clock/1 -> Compare To Constant/1, Lookup Table/1
  Lookup Table/1 -> Out1/1

== system kalmanlib/models/2d Measurement ==
  Clock : Clock
      settings: Decimation=10
  Compare To Constant : simulink/Logic and Bit Operations/Compare To Constant  SystemSampleTime=-1  relop=>=  const=size(zx,2)  LogicOutDataTypeMode=boolean  ZeroCross=off
  Mux : Mux  Inputs=2
  Stop Simulation : Stop
  x : Lookup  InputValues=0:(size(zx,2)-1)  Table=zx'  LookUpMeth=Interpolation-Use End Values  OutDataType=sfix(16)  OutScaling=2^0  SampleTime=tS
  y : Lookup  InputValues=0:(size(zy,2)-1)  Table=zy'  LookUpMeth=Interpolation-Use End Values  OutDataType=sfix(16)  OutScaling=2^0  SampleTime=tS
  z : Outport  OutDataType=sfix(16)  OutScaling=2^0
  wires:
  Clock/1 -> x/1, Compare To Constant/1, y/1
  Compare To Constant/1 -> Stop Simulation/1
  Mux/1 -> z/1
  x/1 -> Mux/1
  y/1 -> Mux/2

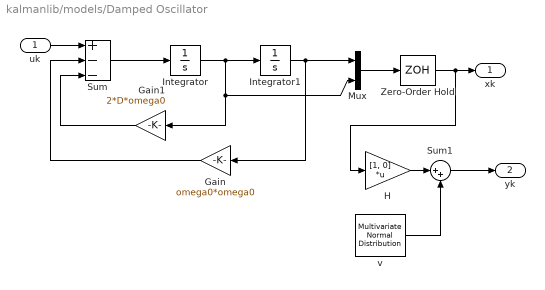
== system kalmanlib/models/Damped Oscillator ==
  uk : Inport  OutDataType=sfix(16)  OutScaling=2^0
  Gain : Gain  Orientation=left  Gain=omega0*omega0  ParameterDataType=sfix(16)  ParameterScaling=2^0  OutDataType=sfix(16)  OutScaling=2^0
  Gain1 : Gain  Orientation=left  Gain=2*D*omega0  ParameterDataType=sfix(16)  ParameterScaling=2^0  OutDataType=sfix(16)  OutScaling=2^0
  H : Gain  Gain=[1, 0]  Multiplication=Matrix(K*u)  ParameterDataType=sfix(16)  ParameterScaling=2^0  OutDataType=sfix(16)  OutScaling=2^0
  Integrator : Integrator
  Integrator1 : Integrator  InitialCondition=1
  Mux : Mux  Inputs=2
  Sum : Sum  Inputs=+--  OutDataType=sfix(16)  OutScaling=2^0
  Sum1 : Sum  Inputs=|++  OutDataType=sfix(16)  OutScaling=2^0
  Zero-Order Hold : ZeroOrderHold  SampleTime=dt
  v : kalmanlib/auxiliary/Multivariate Normal  Distribution  SystemSampleTime=-1  m=0  P=R  seed=seed  tS=dt  C=0
  xk : Outport  OutDataType=sfix(16)  OutScaling=2^0
  yk : Outport  Port=2  OutDataType=sfix(16)  OutScaling=2^0
  wires:
  Sum1/1 -> yk/1
  v/1 -> Sum1/2
  H/1 -> Sum1/1
  Zero-Order Hold/1 -> H/1, xk/1
  uk/1 -> Sum/1
  Gain1/1 -> Sum/3
  Gain/1 -> Sum/2
  Sum/1 -> Integrator/1
  Mux/1 -> Zero-Order Hold/1
  Integrator1/1 -> Mux/1, Gain/1
  Integrator/1 -> Gain1/1, Mux/2, Integrator1/1

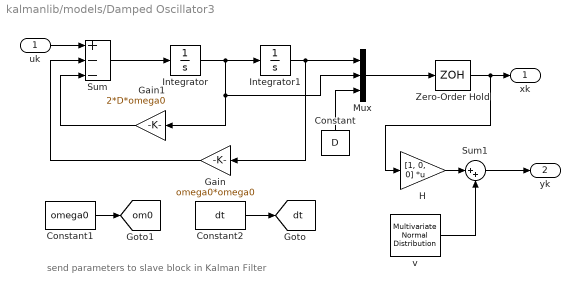
== system kalmanlib/models/Damped Oscillator3 ==
  note: send parameters to slave block
      | in Kalman Filter
  uk : Inport  OutDataType=sfix(16)  OutScaling=2^0
  Constant : Constant  Orientation=up  Value=D  OutDataType=sfix(16)  OutScaling=2^0
  Constant1 : Constant  Value=omega0  OutDataType=sfix(16)  OutScaling=2^0
  Constant2 : Constant  Value=dt  OutDataType=sfix(16)  OutScaling=2^0
  Gain : Gain  Orientation=left  Gain=omega0*omega0  ParameterDataType=sfix(16)  ParameterScaling=2^0  OutDataType=sfix(16)  OutScaling=2^0
  Gain1 : Gain  Orientation=left  Gain=2*D*omega0  ParameterDataType=sfix(16)  ParameterScaling=2^0  OutDataType=sfix(16)  OutScaling=2^0
  H : Gain  Gain=[1, 0, 0]  Multiplication=Matrix(K*u)  ParameterDataType=sfix(16)  ParameterScaling=2^0  OutDataType=sfix(16)  OutScaling=2^0
  Integrator : Integrator
  Integrator1 : Integrator  InitialCondition=1
  Mux : Mux  Inputs=3
  Sum : Sum  Inputs=+--  OutDataType=sfix(16)  OutScaling=2^0
  Sum1 : Sum  Inputs=|++  OutDataType=sfix(16)  OutScaling=2^0
  Zero-Order Hold : ZeroOrderHold  SampleTime=dt
  v : kalmanlib/auxiliary/Multivariate Normal  Distribution  SystemSampleTime=-1  m=0  P=R  seed=seed  tS=dt  C=0
  xk : Outport  OutDataType=sfix(16)  OutScaling=2^0
  yk : Outport  Port=2  OutDataType=sfix(16)  OutScaling=2^0
  tag scope: dt=global, om0=global
  wires:
  Constant2/1 -> [dt]
  Constant1/1 -> [om0]
  Integrator/1 -> Integrator1/1, Gain1/1, Mux/2
  Integrator1/1 -> Gain/1, Mux/1
  Mux/1 -> Zero-Order Hold/1
  Sum/1 -> Integrator/1
  Gain/1 -> Sum/2
  Gain1/1 -> Sum/3
  uk/1 -> Sum/1
  Zero-Order Hold/1 -> xk/1, H/1
  H/1 -> Sum1/1
  v/1 -> Sum1/2
  Sum1/1 -> yk/1
  Constant/1 -> Mux/3

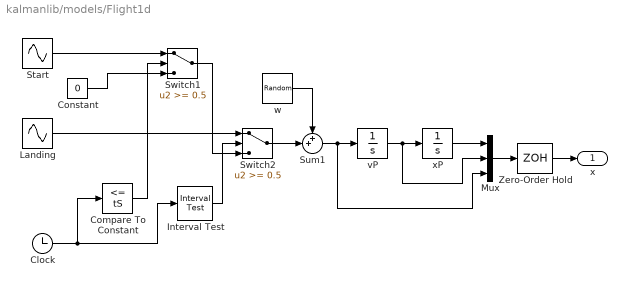
== system kalmanlib/models/Flight1d ==
  Clock : Clock
      settings: Decimation=10
  Compare To Constant : simulink/Logic and Bit Operations/Compare To Constant  SystemSampleTime=-1  relop=<=  const=tS  LogicOutDataTypeMode=boolean  ZeroCross=off
  Constant : Constant  Value=0  OutDataType=sfix(16)  OutScaling=2^0
  Interval Test : simulink/Logic and Bit Operations/Interval Test  SystemSampleTime=-1  IntervalClosedRight=on  uplimit=tS+tF+tL  IntervalClosedLeft=on  lowlimit=tS+tF  LogicOutDataTypeMode=boolean
  Landing : Sin  Amplitude=-v0*pi/(2*tL)  Frequency=pi/tL  Phase=-pi*(tS+tF)/tL  SampleTime=0
  Mux : Mux  Inputs=3
  Start : Sin  Amplitude=v0*pi/(2*tS)  Frequency=pi/tS  SampleTime=0
  Sum1 : Sum  Inputs=++|  OutDataType=sfix(16)  OutScaling=2^0
  Switch1 : Switch  Threshold=0.5
  Switch2 : Switch  Threshold=0.5
  Zero-Order Hold : ZeroOrderHold  SampleTime=dt
  vP : Integrator
  w : RandomNumber  Variance=q  Seed=seed  SampleTime=dt  VectorParams1D=off
  xP : Integrator
  x : Outport  OutDataType=sfix(16)  OutScaling=2^0
  wires:
  Start/1 -> Switch1/1
  Constant/1 -> Switch1/3
  Compare To Constant/1 -> Switch1/2
  Clock/1 -> Compare To Constant/1, Interval Test/1
  Interval Test/1 -> Switch2/2
  Switch1/1 -> Switch2/3
  Landing/1 -> Switch2/1
  vP/1 -> xP/1, Mux/2
  xP/1 -> Mux/1
  Mux/1 -> Zero-Order Hold/1
  Switch2/1 -> Sum1/2
  Sum1/1 -> vP/1, Mux/3
  w/1 -> Sum1/1
  Zero-Order Hold/1 -> x/1

== system kalmanlib/models/Harmonic Oscillator ==
  uk : Inport  OutDataType=sfix(16)  OutScaling=2^0
  Harmonic System : kalmanlib/models/Linear System  SystemSampleTime=-1  A=[cos(w*dt), sin(w*dt)/w; -w*sin(w*dt), cos(w*dt)]  B=[0;1]  H=[1, 0]  Q=[0 0; 0 0]  R=R  x0=[x0; v0]  tS=dt
  x : Outport  OutDataType=sfix(16)  OutScaling=2^0
  y : Outport  Port=2  OutDataType=sfix(16)  OutScaling=2^0
  wires:
  Harmonic System/2 -> y/1
  Harmonic System/1 -> x/1
  uk/1 -> Harmonic System/1

== system kalmanlib/models/Harmonic Oszillator (cont.) ==
  uk : Inport  OutDataType=sfix(16)  OutScaling=2^0
  Gain : Gain  Orientation=left  Gain=omega0*omega0  ParameterDataType=sfix(16)  ParameterScaling=2^0  OutDataType=sfix(16)  OutScaling=2^0
  H : Gain  Gain=[1, 0]  Multiplication=Matrix(K*u)  ParameterDataType=sfix(16)  ParameterScaling=2^0  OutDataType=sfix(16)  OutScaling=2^0
  Integrator : Integrator  InitialCondition=v0
  Integrator1 : Integrator  InitialCondition=x0
  Mux : Mux  Inputs=2
  Sum : Sum  Inputs=+-  OutDataType=sfix(16)  OutScaling=2^0
  Sum1 : Sum  Inputs=|++  OutDataType=sfix(16)  OutScaling=2^0
  Zero-Order Hold : ZeroOrderHold  SampleTime=dt
  v : kalmanlib/auxiliary/Multivariate Normal  Distribution  SystemSampleTime=-1  m=0  P=R  seed=seed  tS=dt  C=0
  xk : Outport  OutDataType=sfix(16)  OutScaling=2^0
  yk : Outport  Port=2  OutDataType=sfix(16)  OutScaling=2^0
  wires:
  Integrator/1 -> Mux/2, Integrator1/1
  Integrator1/1 -> Mux/1, Gain/1
  Mux/1 -> Zero-Order Hold/1
  Sum/1 -> Integrator/1
  Gain/1 -> Sum/2
  uk/1 -> Sum/1
  Zero-Order Hold/1 -> H/1, xk/1
  H/1 -> Sum1/1
  v/1 -> Sum1/2
  Sum1/1 -> yk/1

== system kalmanlib/models/Linear Measurement ==
  x : Inport  OutDataType=sfix(16)  OutScaling=2^0
  H : Gain  Gain=H  Multiplication=Matrix(K*u)  ParameterDataType=sfix(16)  ParameterScaling=2^0  OutDataType=sfix(16)  OutScaling=2^0
  Multivariate Normal  Distribution : kalmanlib/auxiliary/Multivariate Normal  Distribution  SystemSampleTime=-1  m=0  P=R  seed=seed'  tS=dt  C=0
  Sum2 : Sum  Inputs=|++  OutDataType=sfix(16)  OutScaling=2^0
  z : Outport  OutDataType=sfix(16)  OutScaling=2^0
  wires:
  x/1 -> H/1
  Sum2/1 -> z/1
  Multivariate Normal  Distribution/1 -> Sum2/2
  H/1 -> Sum2/1

== system kalmanlib/models/Linear System ==
  uk : Inport  OutDataType=sfix(16)  OutScaling=2^0
  A : Gain  Orientation=left  Gain=A  Multiplication=Matrix(K*u)  ParameterDataType=sfix(16)  ParameterScaling=2^0  OutDataType=sfix(16)  OutScaling=2^0
  B : Gain  Gain=B  Multiplication=Matrix(K*u)  ParameterDataType=sfix(16)  ParameterScaling=2^0  OutDataType=sfix(16)  OutScaling=2^0
  H : Gain  Gain=H  Multiplication=Matrix(K*u)  ParameterDataType=sfix(16)  ParameterScaling=2^0  OutDataType=sfix(16)  OutScaling=2^0
  Sum : Sum  Inputs=||+++  OutDataType=sfix(16)  OutScaling=2^0
  Sum1 : Sum  Inputs=|++  OutDataType=sfix(16)  OutScaling=2^0
  v : kalmanlib/auxiliary/Multivariate Normal  Distribution  SystemSampleTime=-1  m=0  P=R  seed=seed2  tS=tS  C=0
  w : kalmanlib/auxiliary/Multivariate Normal  Distribution  SystemSampleTime=-1  m=0  P=Q  seed=seed1  tS=tS  C=0
  x : UnitDelay  X0=x0  SampleTime=-1
  xk : Outport  OutDataType=sfix(16)  OutScaling=2^0
  zk : Outport  Port=2  OutDataType=sfix(16)  OutScaling=2^0
  wires:
  B/1 -> Sum/2
  A/1 -> Sum/3
  uk/1 -> B/1
  x/1 -> xk/1, A/1, H/1
  Sum/1 -> x/1
  w/1 -> Sum/1
  H/1 -> Sum1/1
  v/1 -> Sum1/2
  Sum1/1 -> zk/1

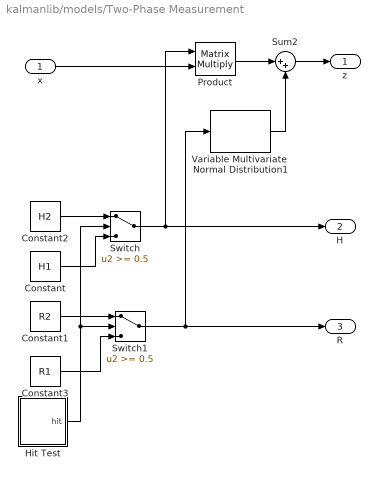
== system kalmanlib/models/Two-Phase Measurement ==
  x : Inport  OutDataType=sfix(16)  OutScaling=2^0
  Constant : Constant  Value=H1  VectorParams1D=off  OutDataType=sfix(16)  OutScaling=2^0
  Constant1 : Constant  Value=R2  VectorParams1D=off  OutDataType=sfix(16)  OutScaling=2^0
  Constant2 : Constant  Value=H2  VectorParams1D=off  OutDataType=sfix(16)  OutScaling=2^0
  Constant3 : Constant  Value=R1  VectorParams1D=off  OutDataType=sfix(16)  OutScaling=2^0
  Hit Test : Subsystem
  Product : Product  Multiplication=Matrix(*)  OutDataType=sfix(16)  OutScaling=2^0  RndMeth=Zero
  Sum2 : Sum  Inputs=|++  OutDataType=sfix(16)  OutScaling=2^0
  Switch : Switch  Threshold=0.5
  Switch1 : Switch  Threshold=0.5
  Variable Multivariate  Normal Distribution1 : kalmanlib/auxiliary/Variable Multivariate  Normal Distribution  SystemSampleTime=-1  m=0  seed=seed'  tS=dt
  z : Outport  OutDataType=sfix(16)  OutScaling=2^0
  H : Outport  Port=2  OutDataType=sfix(16)  OutScaling=2^0
  R : Outport  Port=3  OutDataType=sfix(16)  OutScaling=2^0
  wires:
  Variable Multivariate  Normal Distribution1/1 -> Sum2/2
  Product/1 -> Sum2/1
  Switch1/1 -> Variable Multivariate  Normal Distribution1/1, R/1
  Constant3/1 -> Switch1/3
  Constant1/1 -> Switch1/1
  Constant/1 -> Switch/3
  Constant2/1 -> Switch/1
  Hit Test/1(hit) -> Switch1/2, Switch/2
  Switch/1 -> Product/1, H/1
  x/1 -> Product/2
  Sum2/1 -> z/1

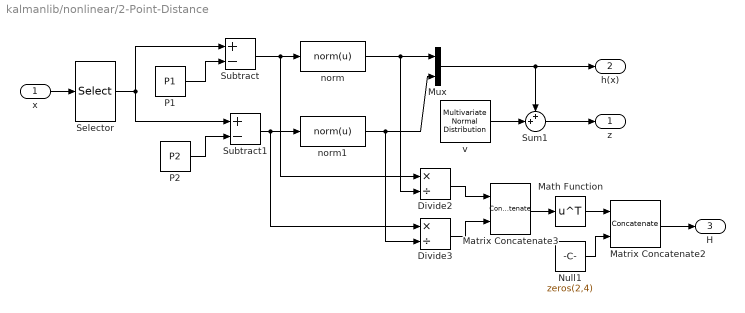
== system kalmanlib/nonlinear/2-Point-Distance ==
  x : Inport  OutDataType=sfix(16)  OutScaling=2^0
  Divide2 : Product  Inputs=*/  OutDataType=sfix(16)  OutScaling=2^-10
  Divide3 : Product  Inputs=*/  OutDataType=sfix(16)  OutScaling=2^-10
  Math Function : Math  Operator=transpose  OutDataType=sfix(16)  OutScaling=2^0  SaturateOnIntegerOverflow=on
  Matrix Concatenate2 : Concatenate  Mode=Multidimensional array  ConcatenateDimension=2
  Matrix Concatenate3 : Concatenate  Mode=Multidimensional array  ConcatenateDimension=2
  Mux : Mux  Inputs=2
  Null1 : Constant  Value=zeros(2,4)  VectorParams1D=off  OutDataType=sfix(16)  OutScaling=2^0
  P1 : Constant  Value=P1  VectorParams1D=off  OutDataType=sfix(16)  OutScaling=2^0
  P2 : Constant  Value=P2  VectorParams1D=off  OutDataType=sfix(16)  OutScaling=2^0
  Selector : Selector  InputPortWidth=6  IndexOptions=Index vector (dialog)  Indices=[1 2]  OutputSizes=1
  Subtract : Sum  Inputs=+-  OutDataType=sfix(16)  OutScaling=2^-10
  Subtract1 : Sum  Inputs=+-  OutDataType=sfix(16)  OutScaling=2^-10
  Sum1 : Sum  Inputs=++|  OutDataType=sfix(16)  OutScaling=2^0
  norm : MATLABFcn  MATLABFcn=norm(u)  OutputDimensions=1
  norm1 : MATLABFcn  MATLABFcn=norm(u)  OutputDimensions=1
  v : kalmanlib/auxiliary/Multivariate Normal  Distribution  SystemSampleTime=-1  m=0  P=R  seed=seed  tS=dt  C=0
  z : Outport  OutDataType=sfix(16)  OutScaling=2^0
  h(x) : Outport  Port=2  OutDataType=sfix(16)  OutScaling=2^0
  H : Outport  Port=3  OutDataType=sfix(16)  OutScaling=2^0
  wires:
  Math Function/1 -> Matrix Concatenate2/1
  v/1 -> Sum1/2
  Sum1/1 -> z/1
  Mux/1 -> h(x)/1, Sum1/1
  x/1 -> Selector/1
  Selector/1 -> Subtract1/1, Subtract/1
  P1/1 -> Subtract/2
  P2/1 -> Subtract1/2
  Subtract/1 -> norm/1, Divide2/1
  Subtract1/1 -> norm1/1, Divide3/1
  norm/1 -> Mux/1, Divide2/2
  norm1/1 -> Mux/2, Divide3/2
  Matrix Concatenate2/1 -> H/1
  Divide2/1 -> Matrix Concatenate3/1
  Divide3/1 -> Matrix Concatenate3/2
  Null1/1 -> Matrix Concatenate2/2
  Matrix Concatenate3/1 -> Math Function/1

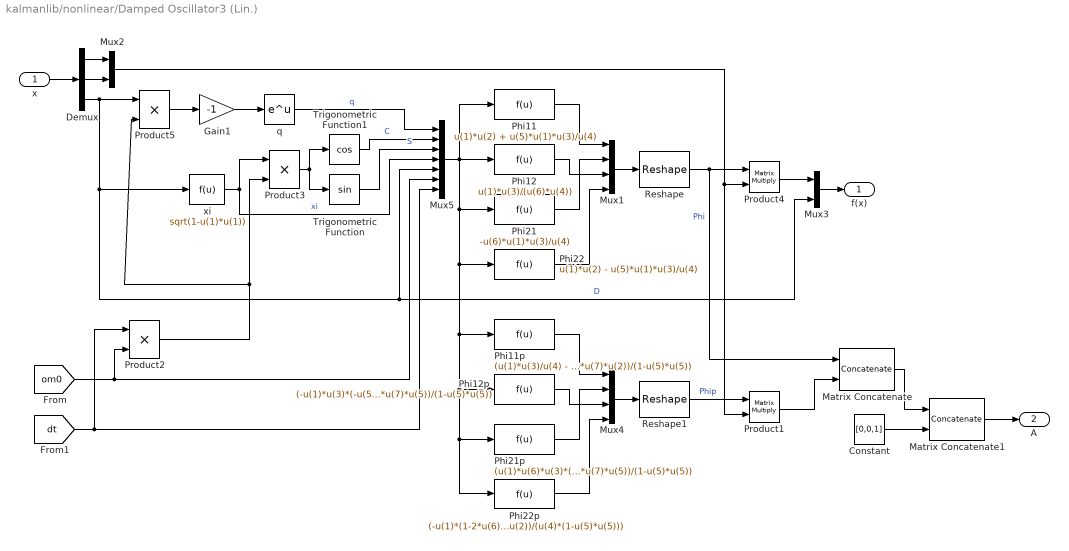
== system kalmanlib/nonlinear/Damped Oscillator3 (Lin.) ==
  x : Inport  OutDataType=sfix(16)  OutScaling=2^0
  Constant : Constant  Value=[0,0,1]  VectorParams1D=off  OutDataType=sfix(16)  OutScaling=2^0
  Demux : Demux  Outputs=3
  Gain1 : Gain  Gain=-1  ParameterDataType=sfix(16)  ParameterScaling=2^0  OutDataType=sfix(16)  OutScaling=2^0
  Matrix Concatenate : Concatenate  Mode=Multidimensional array  ConcatenateDimension=2
  Matrix Concatenate1 : Concatenate  Mode=Multidimensional array
  Mux1 : Mux
  Mux2 : Mux  Inputs=2
  Mux3 : Mux  Inputs=2
  Mux4 : Mux
  Mux5 : Mux  Inputs=7
  Phi11 : Fcn  Expr=u(1)*u(2) + u(5)*u(1)*u(3)/u(4)
  Phi11p : Fcn  Expr=(u(1)*u(3)/u(4) - u(1)*u(6)*u(7)*u(2))/(1-u(5)*u(5))
  Phi12 : Fcn  Expr=u(1)*u(3)/(u(6)*u(4))
  Phi12p : Fcn  Expr=(-u(1)*u(3)*(-u(5)+u(6)*u(7)*(1-u(5)*u(5)))/(u(4)*u(6)) - u(1)*u(2)*u(7)*u(5))/(1-u(5)*u(5))
  Phi21 : Fcn  Expr=-u(6)*u(1)*u(3)/u(4)
  Phi21p : Fcn  Expr=(u(1)*u(6)*u(3)*(-u(5)+u(6)*u(7)*(1-u(5)*u(5)))/u(4) + u(6)*u(6)*u(1)*u(2)*u(7)*u(5))/(1-u(5)*u(5))
  Phi22 : Fcn  Expr=u(1)*u(2) - u(5)*u(1)*u(3)/u(4)
  Phi22p : Fcn  Expr=(-u(1)*(1-2*u(6)*u(7)*u(5)*(1-u(5)*u(5)))*u(3) - u(1)*(-u(4)*u(6)*u(7)+2*u(4)*(1-u(5)*u(5))*u(6)*u(7))*u(2))/(u(4)*(1-u(5)*u(5)))
  Product1 : Product  Multiplication=Matrix(*)  OutDataType=sfix(16)  OutScaling=2^0  RndMeth=Zero
  Product2 : Product  OutDataType=sfix(16)  OutScaling=2^0  RndMeth=Zero
  Product3 : Product  OutDataType=sfix(16)  OutScaling=2^0  RndMeth=Zero
  Product4 : Product  Multiplication=Matrix(*)  OutDataType=sfix(16)  OutScaling=2^0  RndMeth=Zero
  Product5 : Product  OutDataType=sfix(16)  OutScaling=2^0  RndMeth=Zero
  Reshape : Reshape  OutputDimensionality=Customize  OutputDimensions=[2,2]
  Reshape1 : Reshape  OutputDimensionality=Customize  OutputDimensions=[2,2]
  Trigonometric Function : Trigonometry
  Trigonometric Function1 : Trigonometry  Operator=cos
  q : Math  OutDataType=sfix(16)  OutScaling=2^0  SaturateOnIntegerOverflow=on
  xi : Fcn  Expr=sqrt(1-u(1)*u(1))
  f(x) : Outport  OutDataType=sfix(16)  OutScaling=2^0
  A : Outport  Port=2  OutDataType=sfix(16)  OutScaling=2^0
  wires:
  Gain1/1 -> q/1
  Product3/1 -> Trigonometric Function/1, Trigonometric Function1/1
  Product5/1 -> Gain1/1
  Trigonometric Function1/1 -> Mux5/2  "C"
  Product2/1 -> Product5/2, Product3/2
  [dt] -> Product2/1, Mux5/7
  [om0] -> Product2/2, Mux5/6
  Mux3/1 -> f(x)/1
  Product4/1 -> Mux3/1
  Mux2/1 -> Product4/2, Product1/2
  Demux/2 -> Mux2/2
  Demux/1 -> Mux2/1
  Reshape/1 -> Product4/1, Matrix Concatenate/1  "Phi"
  Mux1/1 -> Reshape/1
  xi/1 -> Product3/1, Mux5/4  "xi"
  Demux/3 -> Product5/1, xi/1, Mux3/2, Mux5/5  "D"
  x/1 -> Demux/1
  q/1 -> Mux5/1  "q"
  Trigonometric Function/1 -> Mux5/3  "S"
  Phi11/1 -> Mux1/1
  Mux5/1 -> Phi11/1, Phi12/1, Phi21/1, Phi22/1, Phi11p/1, Phi12p/1, Phi22p/1, Phi21p/1
  Phi21/1 -> Mux1/2
  Phi22/1 -> Mux1/4
  Mux4/1 -> Reshape1/1
  Phi11p/1 -> Mux4/1
  Phi21p/1 -> Mux4/2
  Phi22p/1 -> Mux4/4
  Reshape1/1 -> Product1/1  "Phip"
  Product1/1 -> Matrix Concatenate/2
  Matrix Concatenate/1 -> Matrix Concatenate1/1
  Constant/1 -> Matrix Concatenate1/2
  Matrix Concatenate1/1 -> A/1
  Phi12/1 -> Mux1/3
  Phi12p/1 -> Mux4/3

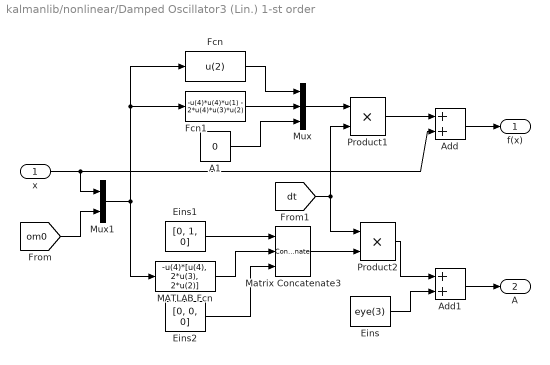
== system kalmanlib/nonlinear/Damped Oscillator3 (Lin.) 1-st order ==
  x : Inport  OutDataType=sfix(16)  OutScaling=2^0
  A1 : Constant  Value=0  OutDataType=sfix(16)  OutScaling=2^0
  Add : Sum  OutDataType=sfix(16)  OutScaling=2^-10
  Add1 : Sum  OutDataType=sfix(16)  OutScaling=2^-10
  Eins : Constant  Value=eye(3)  VectorParams1D=off  OutDataType=sfix(16)  OutScaling=2^0
  Eins1 : Constant  Value=[0, 1, 0]  VectorParams1D=off  OutDataType=sfix(16)  OutScaling=2^0
  Eins2 : Constant  Value=[0, 0, 0]  VectorParams1D=off  OutDataType=sfix(16)  OutScaling=2^0
  Fcn : Fcn  Expr=u(2)
  Fcn1 : Fcn  Expr=-u(4)*u(4)*u(1) - 2*u(4)*u(3)*u(2)
  MATLAB Fcn : MATLABFcn  MATLABFcn=-u(4)*[u(4), 2*u(3), 2*u(2)]  OutputDimensions=[1,3]  Output1D=off
  Matrix Concatenate3 : Concatenate  NumInputs=3  Mode=Multidimensional array
  Mux : Mux  Inputs=3
  Mux1 : Mux  Inputs=2
  Product1 : Product  OutDataType=sfix(16)  OutScaling=2^0  RndMeth=Zero
  Product2 : Product  OutDataType=sfix(16)  OutScaling=2^0  RndMeth=Zero
  f(x) : Outport  OutDataType=sfix(16)  OutScaling=2^0
  A : Outport  Port=2  OutDataType=sfix(16)  OutScaling=2^0
  wires:
  Mux1/1 -> Fcn/1, Fcn1/1, MATLAB Fcn/1
  x/1 -> Mux1/1, Add/2
  [om0] -> Mux1/2
  [dt] -> Product1/2, Product2/1
  Matrix Concatenate3/1 -> Product2/2
  Eins2/1 -> Matrix Concatenate3/3
  MATLAB Fcn/1 -> Matrix Concatenate3/2
  Eins1/1 -> Matrix Concatenate3/1
  Add1/1 -> A/1
  Product2/1 -> Add1/1
  Eins/1 -> Add1/2
  A1/1 -> Mux/3
  Fcn1/1 -> Mux/2
  Fcn/1 -> Mux/1
  Product1/1 -> Add/1
  Add/1 -> f(x)/1
  Mux/1 -> Product1/1

== system kalmanlib/kalman filter/Extended Kalman Filter (Measurement)/K corrector ==
  Pk' : Inport  OutDataType=sfix(16)  OutScaling=2^0
  H : Inport  Port=2  OutDataType=sfix(16)  OutScaling=2^0
  Add : Sum  OutDataType=sfix(16)  OutScaling=2^-10
  Math Function : Math  Operator=transpose  OutDataType=sfix(16)  OutScaling=2^0  SaturateOnIntegerOverflow=on
  Product : Product  Inputs=3  Multiplication=Matrix(*)  OutDataType=sfix(16)  OutScaling=2^0  RndMeth=Zero
  Product1 : Product  Inputs=**/  Multiplication=Matrix(*)  OutDataType=sfix(16)  OutScaling=2^0  RndMeth=Zero
  R : Constant  Value=R  OutDataType=sfix(16)  OutScaling=2^0
  K : Outport  OutDataType=sfix(16)  OutScaling=2^0
  wires:
  Add/1 -> Product1/3
  Product1/1 -> K/1
  H/1 -> Math Function/1, Product/1
  Pk'/1 -> Product1/1, Product/2
  Math Function/1 -> Product1/2, Product/3
  Product/1 -> Add/1
  R/1 -> Add/2

== system kalmanlib/kalman filter/Extended Kalman Filter (Measurement)/Measurement ==
  note: Trivial Measurement
      | z = x
  x : Inport  OutDataType=sfix(16)  OutScaling=2^0
  One : MATLABFcn  MATLABFcn=eye(size(u,1))  Output1D=off
  h(x) : Outport  OutDataType=sfix(16)  OutScaling=2^0
  H : Outport  Port=2  OutDataType=sfix(16)  OutScaling=2^0
  wires:
  x/1 -> One/1, h(x)/1
  One/1 -> H/1

== system kalmanlib/kalman filter/Extended Kalman Filter (Measurement)/P corrector ==
  K : Inport  OutDataType=sfix(16)  OutScaling=2^0
  Pk' : Inport  Port=2  OutDataType=sfix(16)  OutScaling=2^0
  H : Inport  Port=3  OutDataType=sfix(16)  OutScaling=2^0
  Add1 : Sum  Inputs=+-  OutDataType=sfix(16)  OutScaling=2^-10
  Eins : Constant  Value=eye(size(P0))  VectorParams1D=off  OutDataType=sfix(16)  OutScaling=2^0
  Product1 : Product  Multiplication=Matrix(*)  OutDataType=sfix(16)  OutScaling=2^0  RndMeth=Zero
  Product2 : Product  Multiplication=Matrix(*)  OutDataType=sfix(16)  OutScaling=2^0  RndMeth=Zero
  Pk : Outport  OutDataType=sfix(16)  OutScaling=2^0
  wires:
  H/1 -> Product2/2
  K/1 -> Product2/1
  Add1/1 -> Product1/1
  Eins/1 -> Add1/1
  Product2/1 -> Add1/2
  Pk'/1 -> Product1/2
  Product1/1 -> Pk/1

== system kalmanlib/kalman filter/Extended Kalman Filter (Measurement)/P predictor ==
  Pk : Inport  OutDataType=sfix(16)  OutScaling=2^0
  A : Constant  Value=A  OutDataType=sfix(16)  OutScaling=2^0
  A' : Constant  Value=A'  OutDataType=sfix(16)  OutScaling=2^0
  Add : Sum  OutDataType=sfix(16)  OutScaling=2^-10
  Product : Product  Inputs=3  Multiplication=Matrix(*)  OutDataType=sfix(16)  OutScaling=2^0  RndMeth=Zero
  Q : Constant  Value=Q  VectorParams1D=off  OutDataType=sfix(16)  OutScaling=2^0
  Pk' : Outport  OutDataType=sfix(16)  OutScaling=2^0
  wires:
  Add/1 -> Pk'/1
  Q/1 -> Add/2
  Product/1 -> Add/1
  A'/1 -> Product/3
  Pk/1 -> Product/2
  A/1 -> Product/1

== system kalmanlib/kalman filter/Extended Kalman Filter (Measurement)/x corrector ==
  xk' : Inport  OutDataType=sfix(16)  OutScaling=2^0
  zk : Inport  Port=2  OutDataType=sfix(16)  OutScaling=2^0
  K : Inport  Port=3  OutDataType=sfix(16)  OutScaling=2^0
  h(xk') : Inport  Port=4  OutDataType=sfix(16)  OutScaling=2^0
  Add : Sum  OutDataType=sfix(16)  OutScaling=2^-10
  Add1 : Sum  Inputs=-+  OutDataType=sfix(16)  OutScaling=2^-10
  Product1 : Product  Multiplication=Matrix(*)  OutDataType=sfix(16)  OutScaling=2^0  RndMeth=Zero
  x(k+1) : Outport  OutDataType=sfix(16)  OutScaling=2^0
  wires:
  h(xk')/1 -> Add1/1
  Add1/1 -> Product1/2
  zk/1 -> Add1/2
  K/1 -> Product1/1
  Product1/1 -> Add/2
  xk'/1 -> Add/1
  Add/1 -> x(k+1)/1

== system kalmanlib/kalman filter/Extended Kalman Filter (Measurement)/x predictor ==
  xk : Inport  Orientation=left  OutDataType=sfix(16)  OutScaling=2^0
  uk : Inport  Orientation=left  Port=2  OutDataType=sfix(16)  OutScaling=2^0
  Add : Sum  Orientation=left  OutDataType=sfix(16)  OutScaling=2^-10
  Gain : Gain  Orientation=left  Gain=A  Multiplication=Matrix(K*u)  ParameterDataType=sfix(16)  ParameterScaling=2^0  OutDataType=sfix(16)  OutScaling=2^0
  Gain1 : Gain  Orientation=left  Gain=B  Multiplication=Matrix(K*u)  ParameterDataType=sfix(16)  ParameterScaling=2^0  OutDataType=sfix(16)  OutScaling=2^0
  x(k+1)' : Outport  Orientation=left  OutDataType=sfix(16)  OutScaling=2^0
  wires:
  xk/1 -> Gain/1
  uk/1 -> Gain1/1
  Gain/1 -> Add/1
  Gain1/1 -> Add/2
  Add/1 -> x(k+1)'/1

== system kalmanlib/kalman filter/Extended Kalman Filter (System)/K corrector ==
  Pk' : Inport  OutDataType=sfix(16)  OutScaling=2^0
  Add : Sum  OutDataType=sfix(16)  OutScaling=2^-10
  C : Constant  Value=H  VectorParams1D=off  OutDataType=sfix(16)  OutScaling=2^0
  C' : Constant  Value=H'  VectorParams1D=off  OutDataType=sfix(16)  OutScaling=2^0
  Product : Product  Inputs=3  Multiplication=Matrix(*)  OutDataType=sfix(16)  OutScaling=2^0  RndMeth=Zero
  Product1 : Product  Inputs=**/  Multiplication=Matrix(*)  OutDataType=sfix(16)  OutScaling=2^0  RndMeth=Zero
  R : Constant  Value=R  OutDataType=sfix(16)  OutScaling=2^0
  K : Outport  OutDataType=sfix(16)  OutScaling=2^0
  wires:
  C'/1 -> Product/3, Product1/2
  R/1 -> Add/2
  Product/1 -> Add/1
  Pk'/1 -> Product/2, Product1/1
  C/1 -> Product/1
  Product1/1 -> K/1
  Add/1 -> Product1/3
